simulink model "ModeAdjust"  (R2018b)
settings: Solver=FixedStepDiscrete  StartTime=0.0  StopTime=inf  FixedStep=0.01  RelTol=1e-3
undefined symbols (not defined in the file or in its folder): IfKeSMSbSeatMovBkRclnEnable_Val, IfKeSMSbSeatMovFrwdBkwdEnable_Val, IfKeSMSbSeatMovFtrstEnable_Val, IfKeSMSbSeatMovHdrstFrwdBkwdEnable_Val, IfKeSMSbSeatMovHdUpwdDnwdEnable_Val, IfKeSMSbSeatMovLgrstEnable_Val, IfKeSMSbSeatMovLtwdRtwdEnable_Val, IfVeSMSeStNumConfig, KeSMSbArmscreenMovEnable_Val, KeSMSbSeatMovLgrstExpdEnable_Val, KeSMSuFirstRwStBackPosDelta_Val, KeSMSuFirstRwStBackPosTolr_Val, KeSMSuFirstRwStCushFrntPosDelta_Val, KeSMSuFirstRwStCushFrntPosTolr_Val, KeSMSuFirstRwStCushRePosDelta_Val, KeSMSuFirstRwStCushRePosTolr_Val, KeSMSuFirstRwStFootrestPosDelta_Val, KeSMSuFirstRwStFootrestPosTolr_Val, KeSMSuFirstRwStFwdBkwdPosDelta_Val, KeSMSuFirstRwStFwdBkwdPosTolr_Val, KeSMSuMdMotFinshdTm_Val, KeSMSuMdRetryTm1_Val, KeSMSuModeReqDurgTm_Val, KeSMSuSecRwStArmTochPosDelta_Val, KeSMSuSecRwStArmTochPosTolr_Val, KeSMSuSecRwStBackPosDelta_Val, KeSMSuSecRwStBackPosTolr_Val, KeSMSuSecRwStFtrstUpwdDnwdPosDelta_Val, KeSMSuSecRwStFtrstUpwdDnwdPosTolr_Val, KeSMSuSecRwStFwdBkwdPosDelta_Val, KeSMSuSecRwStFwdBkwdPosTolr_Val, KeSMSuSecRwStHeadrestFwdBkwdPosDelta_Val, KeSMSuSecRwStHeadrestFwdBkwdPosTolr_Val, KeSMSuSecRwStHeadrestUpwdDwnwdPosDelta_Val, KeSMSuSecRwStHeadrestUpwdDwnwdPosTolr_Val, KeSMSuSecRwStLegrestInOutPosDelta_Val, KeSMSuSecRwStLegrestInOutPosTolr_Val, KeSMSuSecRwStLegrestUpwdDwnwdPosDelta_Val, KeSMSuSecRwStLegrestUpwdDwnwdPosTolr_Val, KeSMSuSecRwStLwdRwdPosDelta_Val, KeSMSuSecRwStLwdRwdPosTolr_Val, KeSMSuSecRwStVIPFtrstRefAngle_Val, KeSMSuThirdRwStFwdBkwdPosDelta_Val, KeSMSuThirdRwStFwdBkwdPosTolr_Val, KeSMSuThrdRwCushFoldPosDelta_Val, KeSMSuThrdRwCushFoldPosTolr_Val, KeSMSuThrdRwStBackPosDelta_Val, KeSMSuThrdRwStBackPosTolr_Val, KeSMSw4SLegrstCloseMdSecRwLtStFtrstUpwdDnwdPos_Val, KeSMSw4SLegrstCloseMdSecRwLtStFtrstUpwdDnwdPosMax_Val, KeSMSw4SLegrstCloseMdSecRwLtStFtrstUpwdDnwdPosMin_Val, KeSMSw4SLegrstCloseMdSecRwLtStLgrstOtwdInwdPos_Val, KeSMSw4SLegrstCloseMdSecRwLtStLgrstOtwdInwdPosMax_Val, KeSMSw4SLegrstCloseMdSecRwLtStLgrstOtwdInwdPosMin_Val, KeSMSw4SLegrstCloseMdSecRwLtStLgrstUpwdDnwdPos_Val, KeSMSw4SLegrstCloseMdSecRwLtStLgrstUpwdDnwdPosMax_Val, KeSMSw4SLegrstCloseMdSecRwLtStLgrstUpwdDnwdPosMin_Val, KeSMSw4SLegrstCloseMdSecRwRtStFtrstUpwdDnwdPos_Val, KeSMSw4SLegrstCloseMdSecRwRtStFtrstUpwdDnwdPosMax_Val, KeSMSw4SLegrstCloseMdSecRwRtStFtrstUpwdDnwdPosMin_Val ... (+1138)
libraries: Lib x401
(part 2 of 35)

== system ModeAdjust/ModeAdjustRunnable_sys ==
  IfVeSMSeSecRwLtStChldLkRsp_Val_read : Inport
  IfVeSMSeSecRwRtStChldLkRsp_Val_read : Inport  Port=2
  IfVeSMSuDrvStBkReclnUpwdDnwdPos_Val_read : Inport  Port=3
  IfVeSMSuDrvStBkReclnUpwdDnwdPosV_Val_read : Inport  Port=4
  IfVeSMSuDrvStCshnFrntUpwdDnwdPos_Val_read : Inport  Port=5
  IfVeSMSuDrvStCshnFrntUpwdDnwdPosV_Val_read : Inport  Port=6
  IfVeSMSuDrvStCshnRrUpwdDnwdPos_Val_read : Inport  Port=7
  IfVeSMSuDrvStCshnRrUpwdDnwdPosV_Val_read : Inport  Port=8
  IfVeSMSuDrvStFrwdBkwdPos_Val_read : Inport  Port=9
  IfVeSMSuDrvStFrwdBkwdPosV_Val_read : Inport  Port=10
  IfVeSMSuDrvStFtUpwdDnwdPos_Val_read : Inport  Port=11
  IfVeSMSuDrvStFtUpwdDnwdPosV_Val_read : Inport  Port=12
  IfVeSMSuPassStBkReclnUpwdDnwdPos_Val_read : Inport  Port=13
  IfVeSMSuPassStBkReclnUpwdDnwdPosV_Val_read : Inport  Port=14
  IfVeSMSuPassStCshnFrntUpwdDnwdPos_Val_read : Inport  Port=15
  IfVeSMSuPassStCshnFrntUpwdDnwdPosV_Val_read : Inport  Port=16
  IfVeSMSuPassStCshnRrUpwdDnwdPos_Val_read : Inport  Port=17
  IfVeSMSuPassStCshnRrUpwdDnwdPosV_Val_read : Inport  Port=18
  IfVeSMSuPassStFrwdBkwdPos_Val_read : Inport  Port=19
  IfVeSMSuPassStFrwdBkwdPosV_Val_read : Inport  Port=20
  IfVeSMSuPassStFtUpwdDnwdPos_Val_read : Inport  Port=21
  IfVeSMSuPassStFtUpwdDnwdPosV_Val_read : Inport  Port=22
  IfVeSMSuSecRwLtStArmScrnPos_Val_read : Inport  Port=23
  IfVeSMSuSecRwLtStArmScrnPosV_Val_read : Inport  Port=24
  IfVeSMSuSecRwLtStBkReclnUpwdDnwdPos_Val_read : Inport  Port=25
  IfVeSMSuSecRwLtStBkReclnUpwdDnwdPosV_Val_read : Inport  Port=26
  IfVeSMSuSecRwLtStFrwdBkwdPos_Val_read : Inport  Port=27
  IfVeSMSuSecRwLtStFrwdBkwdPosV_Val_read : Inport  Port=28
  IfVeSMSuSecRwLtStHdrstUpwdDnwdPos_Val_read : Inport  Port=29
  IfVeSMSuSecRwLtStHdrstUpwdDnwdPosV_Val_read : Inport  Port=30
  IfVeSMSuSecRwLtStLgrstUpwdDnwdPos_Val_read : Inport  Port=31
  IfVeSMSuSecRwLtStLgrstUpwdDnwdPosV_Val_read : Inport  Port=32
  IfVeSMSuSecRwLtStLtwdRtwdPos_Val_read : Inport  Port=33
  IfVeSMSuSecRwLtStLtwdRtwdPosV_Val_read : Inport  Port=34
  IfVeSMSuSecRwRtStArmScrnPos_Val_read : Inport  Port=35
  IfVeSMSuSecRwRtStArmScrnPosV_Val_read : Inport  Port=36
  IfVeSMSuSecRwRtStBkReclnUpwdDnwdPos_Val_read : Inport  Port=37
  IfVeSMSuSecRwRtStBkReclnUpwdDnwdPosV_Val_read : Inport  Port=38
  IfVeSMSuSecRwRtStFrwdBkwdPos_Val_read : Inport  Port=39
  IfVeSMSuSecRwRtStFrwdBkwdPosV_Val_read : Inport  Port=40
  IfVeSMSuSecRwRtStHdrstUpwdDnwdPos_Val_read : Inport  Port=41
  IfVeSMSuSecRwRtStHPassStUpwdDnwdPosV_Val_read : Inport  Port=42
  IfVeSMSuSecRwRtStLgrstUpwdDnwdPos_Val_read : Inport  Port=43
  IfVeSMSuSecRwRtStLgrstUpwdDnwdPosV_Val_read : Inport  Port=44
  IfVeSMSuSecRwRtStLtwdRtwdPos_Val_read : Inport  Port=45
  IfVeSMSuSecRwRtStLtwdRtwdPosV_Val_read : Inport  Port=46
  IfVeSMSuThdRwLtStBkReclnUpwdDnwdPos_Val_read : Inport  Port=47
  IfVeSMSuThdRwLtStBkReclnUpwdDnwdPosV_Val_read : Inport  Port=48
  IfVeSMSuThdRwLtStCshnFldUpwdDnwdPos_Val_read : Inport  Port=49
  IfVeSMSuThdRwLtStCshnFldUpwdDnwdPosV_Val_read : Inport  Port=50
  IfVeSMSuThdRwLtStFrwdBkwdPos_Val_read : Inport  Port=51
  IfVeSMSuThdRwLtStFrwdBkwdPosV_Val_read : Inport  Port=52
  IfVeSMSuThdRwRStFrwdBkwdPos_Val_read : Inport  Port=53
  IfVeSMSuThdRwRtStBkReclnUpwdDnwdPos_Val_read : Inport  Port=54
  IfVeSMSuThdRwRtStBkReclnUpwdDnwdPosV_Val_read : Inport  Port=55
  IfVeSMSuThdRwRtStCshnFldUpwdDnwdPos_Val_read : Inport  Port=56
  IfVeSMSuThdRwRtStCshnFldUpwdDnwdPosV_Val_read : Inport  Port=57
  IfVeSMSuThdRwRtStFrwdBkwdPosV_Val_read : Inport  Port=58
  IfVeSMSeNotThdRowRtSeaOccStat_Val_read : Inport  Port=59
  IfVeSMSeNotThdRwCtStOccStat_Val_read : Inport  Port=60
  IfVeSMSeNotThdRwLtStOccStat_Val_read : Inport  Port=61
  modestate32_Val_read : Inport  Port=62
  PwrMdChked_Val_read : Inport  Port=63
  IfVeSMSbDrvStBkReclnUpwdDnwdMovConfig_Val_read : Inport  Port=64
  IfVeSMSbDrvStFrwdBkwdMovConfig_Val_read : Inport  Port=65
  IfVeSMSbDrvStFtUpwdDnwdMovConfig_Val_read : Inport  Port=66
  IfVeSMSbPassStBkReclnUpwdDnwdMovConfig_Val_read : Inport  Port=67
  IfVeSMSbPassStFrwdBkwdMovConfig_Val_read : Inport  Port=68
  IfVeSMSbPassStFtUpwdDnwdMovConfig_Val_read : Inport  Port=69
  IfVeSMSbSecRwRtStBkReclnUpwdDnwdMovConfig_Val_read : Inport  Port=70
  IfVeSMSbSecRwRtStBlstOtwdInwdMovConfig_Val_read : Inport  Port=71
  IfVeSMSbSecRwRtStFrwdBkwdMovConfig_Val_read : Inport  Port=72
  IfVeSMSbSecRwRtStLgrstUpwdMovConfig_Val_read : Inport  Port=73
  IfVeSMSbSecRwRtStLtwdRtwdMovConfig_Val_read : Inport  Port=74
  IfVeSMSbThdRwLtStBkReclnUpwdDnwdMovConfig_Val_read : Inport  Port=75
  IfVeSMSbThdRwLtStCshnFldUpwdDnwdMovConfig_Val_read : Inport  Port=76
  IfVeSMSbThdRwLtStFrwdBkwdMovConfig_Val_read : Inport  Port=77
  IfVeSMSbThdRwRtStBkReclnUpwdDnwdMovConfig_Val_read : Inport  Port=78
  IfVeSMSbThdRwRtStCshnFldUpwdDnwdMovConfig_Val_read : Inport  Port=79
  IfVeSMSbThdRwRtStFrwdBkwdMovConfig_Val_read : Inport  Port=80
  IfVeSMSuRrLtStFtUpwdDnwdPos_Val_read : Inport  Port=81
  IfVeSMSuRrLtStFtUpwdDnwdPosV_Val_read : Inport  Port=82
  IfVeSMSuRrRtStFtUpwdDnwdPos_Val_read : Inport  Port=83
  IfVeSMSuRrRtStFtUpwdDnwdPosV_Val_read : Inport  Port=84
  IfVeSMSuSecRwLtStLgrstOtwdInwdPos_Val_read : Inport  Port=85
  IfVeSMSuSecRwLtStLgrstOtwdInwdPosV_Val_read : Inport  Port=86
  IfVeSMSuSecRwRtStLgrstOtwdInwdPos_Val_read : Inport  Port=87
  IfVeSMSuSecRwRtStLgrstOtwdInwdPosV_Val_read : Inport  Port=88
  IfVeSMSbSecRwRtSLgrstExpdMovConfig_Val_read : Inport  Port=89
  IfVeSMSbSecRwRtStFtrstMovConfig_Val_read : Inport  Port=90
  IfVeSMSbSecRwRtStHdUpwdDnwdMovConfig_Val_read : Inport  Port=91
  IfVeSMSbThdRwLtStFrwdCmdSrv_Val_read : Inport  Port=92
  IfVeSMSbThdRwRtStFrwdCmdSrv_Val_read : Inport  Port=93
  IfVeSMSbSecRwRtStHdrstFrwdBkwdMovConfig_Val_read : Inport  Port=94
  IfVeSMSuSecRwLtStHdrstFrwdBkwdPos_Val_read : Inport  Port=95
  IfVeSMSuSecRwLtStHdrstFrwdBkwdPosV_Val_read : Inport  Port=96
  IfVeSMSuSecRwRtStHdrstFrwdBkwdPos_Val_read : Inport  Port=97
  IfVeSMSuSecRwRtStHdrstFrwdBkwdPosV_Val_read : Inport  Port=98
  IfVeSMSeNotSecRowLeSeaOccStat_Val_read : Inport  Port=99
  IfVeSMSeNotSecRowRtSeaOccStat_Val_read : Inport  Port=100
  IfVeSMSeStNumConfig_Val_read : Inport  Port=101
  function : TriggerPort  TriggerType=function-call  VariantControl=(inherit)  SampleTimeType=periodic  SampleTime=-1
  ModeAdjust : Subsystem
  IfVeSMSbDrvStRclCmdSrv_Val_write : Outport
  IfVeSMSbSecRwRtStRclCmdSrv_Val_write : Outport  Port=2
  IfVeSMSbThdRwLtStRclCmdSrv_Val_write : Outport  Port=3
  IfVeSMSbThdRwRtStRclCmdSrv_Val_write : Outport  Port=4
  IfVeSMSuDrvStBkReclnUpwdDnwdTrgtPos_Val_write : Outport  Port=5
  IfVeSMSuDrvStCshnFrntUpwdDnwdTrgtPos_Val_write : Outport  Port=6
  IfVeSMSuDrvStCshnRrUpwdDnwdTrgtPos_Val_write : Outport  Port=7
  IfVeSMSuDrvStFrwdBkwdTrgtPos_Val_write : Outport  Port=8
  IfVeSMSuDrvStFtUpwdDnwdTrgtPos_Val_write : Outport  Port=9
  IfVeSMSuPassStBkReclnUpwdDnwdTrgtPos_Val_write : Outport  Port=10
  IfVeSMSuPassStCshnFrntUpwdDnwdTrgtPos_Val_write : Outport  Port=11
  IfVeSMSuPassStCshnRrUpwdDnwdTrgtPos_Val_write : Outport  Port=12
  IfVeSMSuPassStFrwdBkwdTrgtPos_Val_write : Outport  Port=13
  IfVeSMSuPassStFtUpwdDnwdTrgtPos_Val_write : Outport  Port=14
  IfVeSMSuPassStRclCmdSrv_Val_write : Outport  Port=15
  IfVeSMSuSecRwLtStBkReclnUpwdDnwdTrgtPos_Val_write : Outport  Port=16
  IfVeSMSuSecRwLtStFrwdBkwdTrgtPos_Val_write : Outport  Port=17
  IfVeSMSuSecRwLtStHdrstUpwdDnwdTrgtPos_Val_write : Outport  Port=18
  IfVeSMSuSecRwLtStLgrstUpwdDnwdTrgtPos_Val_write : Outport  Port=19
  IfVeSMSuSecRwLtStLtwdRtwdTrgtPos_Val_write : Outport  Port=20
  IfVeSMSuSecRwLtStRclCmdSrv_Val_write : Outport  Port=21
  IfVeSMSuSecRwRtStBkReclnUpwdDnwdTrgtPos_Val_write : Outport  Port=22
  IfVeSMSuSecRwRtStFrwdBkwdTrgtPos_Val_write : Outport  Port=23
  IfVeSMSuSecRwRtStHdrstUpwdDnwdTrgtPos_Val_write : Outport  Port=24
  IfVeSMSuSecRwRtStLgrstUpwdDnwdTrgtPos_Val_write : Outport  Port=25
  IfVeSMSuSecRwRtStLtwdRtwdTrgtPos_Val_write : Outport  Port=26
  IfVeSMSuThdRwLtStBkReclnUpwdDnwdTrgtPos_Val_write : Outport  Port=27
  IfVeSMSuThdRwLtStCshnFldUpwdDnwdTrgtPos_Val_write : Outport  Port=28
  IfVeSMSuThdRwLtStFrwdBkwdTrgtPos_Val_write : Outport  Port=29
  IfVeSMSuThdRwRtStBkReclnUpwdDnwdTrgtPos_Val_write : Outport  Port=30
  IfVeSMSuThdRwRtStCshnFldUpwdDnwdTrgtPos_Val_write : Outport  Port=31
  IfVeSMSuThdRwRtStFrwdBkwdTrgtPos_Val_write : Outport  Port=32
  isAcsMdEntryArrivedAtTargetPos_Val_write : Outport  Port=33
  isAcsMdEntryDoneFailed_Val_write : Outport  Port=34
  isAcsMdEntryDoneOK_Val_write : Outport  Port=35
  isAcsMdExtArrivedAtTargetPos_Val_write : Outport  Port=36
  isAcsMdExtDoneFailed_Val_write : Outport  Port=37
  isAcsMdExtDoneOK_Val_write : Outport  Port=38
  isLfLugArrivedAtTargetPos_Val_write : Outport  Port=39
  isLfLugDoneFailed_Val_write : Outport  Port=40
  isLfLugDoneOK_Val_write : Outport  Port=41
  isLfRecoveryArrivedAtTargetPos_Val_write : Outport  Port=42
  isLfRecoveryDoneFailed_Val_write : Outport  Port=43
  isLfRecoveryDoneOK_Val_write : Outport  Port=44
  isLfVipArrivedAtTargetPos_Val_write : Outport  Port=45
  isLfVipDoneFailed_Val_write : Outport  Port=46
  isLfVipDoneOK_Val_write : Outport  Port=47
  isRtLugArrivedAtTargetPos_Val_write : Outport  Port=48
  isRtLugDoneFailed_Val_write : Outport  Port=49
  isRtLugDoneOK_Val_write : Outport  Port=50
  isRtRecoveryArrivedAtTargetPos_Val_write : Outport  Port=51
  isRtRecoveryDoneFailed_Val_write : Outport  Port=52
  isRtRecoveryDoneOK_Val_write : Outport  Port=53
  isRtVipArrivedAtTargetPos_Val_write : Outport  Port=54
  isRtVipDoneFailed_Val_write : Outport  Port=55
  isRtVipDoneOK_Val_write : Outport  Port=56
  IfVeSMSuSecRwLtStArmScrnTrgtPos_Val_write : Outport  Port=57
  IfVeSMSuSecRwRtStArmScrnTrgtPos_Val_write : Outport  Port=58
  IfVeSMSuRrLtStFtUpwdDnwdTrgtPos_Val_write : Outport  Port=59
      settings: EnsureOutportIsVirtual=on
  IfVeSMSuRrRtStFtUpwdDnwdTrgtPos_Val_write : Outport  Port=60
      settings: EnsureOutportIsVirtual=on
  IfVeSMSuSecRwLtStLgrstOtwdInwdTrgtPos_Val_write : Outport  Port=61
      settings: EnsureOutportIsVirtual=on
  IfVeSMSuSecRwRtStLgrstOtwdInwdTrgtPos_Val_write : Outport  Port=62
      settings: EnsureOutportIsVirtual=on
  isINTMArrivedAtTargetPos_Val_write : Outport  Port=63
      settings: EnsureOutportIsVirtual=on
  isINTMDoneFailed_Val_write : Outport  Port=64
      settings: EnsureOutportIsVirtual=on
  isINTMDoneOK_Val_write : Outport  Port=65
      settings: EnsureOutportIsVirtual=on
  isLfFamlyArrivedAtTargetPos_Val_write : Outport  Port=66
      settings: EnsureOutportIsVirtual=on
  isLfFamlyDoneFailed_Val_write : Outport  Port=67
      settings: EnsureOutportIsVirtual=on
  isLfFamlyDoneOK_Val_write : Outport  Port=68
      settings: EnsureOutportIsVirtual=on
  isLfLyArrivedAtTargetPos_Val_write : Outport  Port=69
      settings: EnsureOutportIsVirtual=on
  isLfLyDoneFailed_Val_write : Outport  Port=70
      settings: EnsureOutportIsVirtual=on
  isLfLyDoneOK_Val_write : Outport  Port=71
      settings: EnsureOutportIsVirtual=on
  isRfFamlyDoneFailed_Val_write : Outport  Port=72
      settings: EnsureOutportIsVirtual=on
  isRfFamlyDoneOK_Val_write : Outport  Port=73
      settings: EnsureOutportIsVirtual=on
  isRtFamlyArrivedAtTargetPos_Val_write : Outport  Port=74
      settings: EnsureOutportIsVirtual=on
  isRtLyArrivedAtTargetPos_Val_write : Outport  Port=75
      settings: EnsureOutportIsVirtual=on
  isRtLyDoneFailed_Val_write : Outport  Port=76
      settings: EnsureOutportIsVirtual=on
  isRtLyDoneOK_Val_write : Outport  Port=77
      settings: EnsureOutportIsVirtual=on
  IfVeSMSuSecRwLtStHdrstFrwdBkwdTrgtPos_Val_write : Outport  Port=78
      settings: EnsureOutportIsVirtual=on
  IfVeSMSuSecRwRtStHdrstFrwdBkwdTrgtPos_Val_write : Outport  Port=79
      settings: EnsureOutportIsVirtual=on
  IfVeSMSeSecRwLtStMdRclLgSldSpdCrl_Val_write : Outport  Port=80
      settings: EnsureOutportIsVirtual=on
  IfVeSMSeSecRwRtStMdRclLgSldSpdCrl_Val_write : Outport  Port=81
      settings: EnsureOutportIsVirtual=on
  IfVeSMSeThdRwLtStMdRclLgSldSpdCrl_Val_write : Outport  Port=82
      settings: EnsureOutportIsVirtual=on
  IfVeSMSeThdRwRtStMdRclLgSldSpdCrl_Val_write : Outport  Port=83
      settings: EnsureOutportIsVirtual=on
  isINTMRArrivedAtTargetPos_Val_write : Outport  Port=84
      settings: EnsureOutportIsVirtual=on
  isINTMRDoneFailed_Val_write : Outport  Port=85
      settings: EnsureOutportIsVirtual=on
  isINTMRDoneOK_Val_write : Outport  Port=86
      settings: EnsureOutportIsVirtual=on
  isLgrstCloseLArrivedAtTargetPos_Val_write : Outport  Port=87
      settings: EnsureOutportIsVirtual=on
  isLgrstCloseLDoneFailed_Val_write : Outport  Port=88
      settings: EnsureOutportIsVirtual=on
  isLgrstCloseLDoneOK_Val_write : Outport  Port=89
      settings: EnsureOutportIsVirtual=on
  isLgrstCloseRArrivedAtTargetPos_Val_write : Outport  Port=90
      settings: EnsureOutportIsVirtual=on
  isLgrstCloseRDoneFailed_Val_write : Outport  Port=91
      settings: EnsureOutportIsVirtual=on
  isLgrstCloseRDoneOK_Val_write : Outport  Port=92
      settings: EnsureOutportIsVirtual=on
  isLgrstOpenLArrivedAtTargetPos_Val_write : Outport  Port=93
      settings: EnsureOutportIsVirtual=on
  isLgrstOpenLDoneFailed_Val_write : Outport  Port=94
      settings: EnsureOutportIsVirtual=on
  isLgrstOpenLDoneOK_Val_write : Outport  Port=95
      settings: EnsureOutportIsVirtual=on
  isLgrstOpenRArrivedAtTargetPos_Val_write : Outport  Port=96
      settings: EnsureOutportIsVirtual=on
  isLgrstOpenRDoneFailed_Val_write : Outport  Port=97
      settings: EnsureOutportIsVirtual=on
  isLgrstOpenRDoneOK_Val_write : Outport  Port=98
      settings: EnsureOutportIsVirtual=on
  wires:
  IfVeSMSuPassStBkReclnUpwdDnwdPos_Val_read/1 -> ModeAdjust/3(IfVeSMSuPassStBkReclnUpwdDnwdPos_Val_read)
  IfVeSMSuPassStBkReclnUpwdDnwdPosV_Val_read/1 -> ModeAdjust/4(IfVeSMSuPassStBkReclnUpwdDnwdPosV_Val_read)
  IfVeSMSuPassStCshnFrntUpwdDnwdPos_Val_read/1 -> ModeAdjust/5(IfVeSMSuPassStCshnFrntUpwdDnwdPos_Val_read)
  IfVeSMSuPassStCshnFrntUpwdDnwdPosV_Val_read/1 -> ModeAdjust/6(IfVeSMSuPassStCshnFrntUpwdDnwdPosV_Val_read)
  IfVeSMSuPassStCshnRrUpwdDnwdPos_Val_read/1 -> ModeAdjust/7(IfVeSMSuPassStCshnRrUpwdDnwdPos_Val_read)
  IfVeSMSuPassStCshnRrUpwdDnwdPosV_Val_read/1 -> ModeAdjust/8(IfVeSMSuPassStCshnRrUpwdDnwdPosV_Val_read)
  IfVeSMSuPassStFrwdBkwdPos_Val_read/1 -> ModeAdjust/9(IfVeSMSuPassStFrwdBkwdPos_Val_read)
  IfVeSMSuPassStFrwdBkwdPosV_Val_read/1 -> ModeAdjust/10(IfVeSMSuPassStFrwdBkwdPosV_Val_read)
  IfVeSMSuPassStFtUpwdDnwdPos_Val_read/1 -> ModeAdjust/11(IfVeSMSuPassStFtUpwdDnwdPos_Val_read)
  IfVeSMSuPassStFtUpwdDnwdPosV_Val_read/1 -> ModeAdjust/12(IfVeSMSuPassStFtUpwdDnwdPosV_Val_read)
  IfVeSMSuSecRwLtStArmScrnPos_Val_read/1 -> ModeAdjust/58(IfVeSMSuSecRwLtStArmScrnPos_Val_read)
  IfVeSMSuSecRwLtStArmScrnPosV_Val_read/1 -> ModeAdjust/59(IfVeSMSuSecRwLtStArmScrnPosV_Val_read)
  IfVeSMSuSecRwLtStBkReclnUpwdDnwdPos_Val_read/1 -> ModeAdjust/13(IfVeSMSuSecRwLtStBkReclnUpwdDnwdPos_Val_read)
  IfVeSMSuSecRwLtStBkReclnUpwdDnwdPosV_Val_read/1 -> ModeAdjust/14(IfVeSMSuSecRwLtStBkReclnUpwdDnwdPosV_Val_read)
  IfVeSMSuSecRwLtStFrwdBkwdPos_Val_read/1 -> ModeAdjust/15(IfVeSMSuSecRwLtStFrwdBkwdPos_Val_read)
  IfVeSMSuSecRwLtStFrwdBkwdPosV_Val_read/1 -> ModeAdjust/16(IfVeSMSuSecRwLtStFrwdBkwdPosV_Val_read)
  IfVeSMSuSecRwLtStLgrstUpwdDnwdPos_Val_read/1 -> ModeAdjust/19(IfVeSMSuSecRwLtStLgrstUpwdDnwdPos_Val_read)
  IfVeSMSuSecRwLtStLgrstUpwdDnwdPosV_Val_read/1 -> ModeAdjust/20(IfVeSMSuSecRwLtStLgrstUpwdDnwdPosV_Val_read)
  IfVeSMSuSecRwLtStLtwdRtwdPos_Val_read/1 -> ModeAdjust/21(IfVeSMSuSecRwLtStLtwdRtwdPos_Val_read)
  IfVeSMSuSecRwLtStLtwdRtwdPosV_Val_read/1 -> ModeAdjust/22(IfVeSMSuSecRwLtStLtwdRtwdPosV_Val_read)
  IfVeSMSuSecRwRtStArmScrnPos_Val_read/1 -> ModeAdjust/60(SecRwRtStArmScrnPos_Val_read)
  IfVeSMSuSecRwRtStArmScrnPosV_Val_read/1 -> ModeAdjust/61(SecRwRtStArmScrnPosV_Val_read)
  IfVeSMSuSecRwRtStBkReclnUpwdDnwdPos_Val_read/1 -> ModeAdjust/35(IfVeSMSuSecRwRtStBkReclnUpwdDnwdPos_Val_read)
  IfVeSMSuSecRwRtStBkReclnUpwdDnwdPosV_Val_read/1 -> ModeAdjust/36(IfVeSMSuSecRwRtStBkReclnUpwdDnwdPosV_Val_read)
  IfVeSMSuSecRwRtStFrwdBkwdPos_Val_read/1 -> ModeAdjust/37(IfVeSMSuSecRwRtStFrwdBkwdPos_Val_read)
  IfVeSMSuSecRwRtStFrwdBkwdPosV_Val_read/1 -> ModeAdjust/38(IfVeSMSuSecRwRtStFrwdBkwdPosV_Val_read)
  IfVeSMSuSecRwRtStHdrstUpwdDnwdPos_Val_read/1 -> ModeAdjust/39(IfVeSMSuSecRwRtStHPassStUpwdDnwdPos_Val_read)
  IfVeSMSuSecRwRtStHPassStUpwdDnwdPosV_Val_read/1 -> ModeAdjust/40(IfVeSMSuSecRwRtStHPassStUpwdDnwdPosV_Val_read)
  IfVeSMSuSecRwRtStLgrstUpwdDnwdPos_Val_read/1 -> ModeAdjust/41(IfVeSMSuSecRwRtStLgrstUpwdDnwdPos_Val_read)
  IfVeSMSuSecRwRtStLgrstUpwdDnwdPosV_Val_read/1 -> ModeAdjust/42(IfVeSMSuSecRwRtStLgrstUpwdDnwdPosV_Val_read)
  IfVeSMSuSecRwRtStLtwdRtwdPos_Val_read/1 -> ModeAdjust/43(IfVeSMSuSecRwRtStLtwdRtwdPos_Val_read)
  IfVeSMSuSecRwRtStLtwdRtwdPosV_Val_read/1 -> ModeAdjust/44(IfVeSMSuSecRwRtStLtwdRtwdPosV_Val_read)
  IfVeSMSuThdRwLtStBkReclnUpwdDnwdPos_Val_read/1 -> ModeAdjust/23(IfVeSMSuThdRwLtStBkReclnUpwdDnwdPos_Val_read)
  IfVeSMSuThdRwLtStBkReclnUpwdDnwdPosV_Val_read/1 -> ModeAdjust/24(IfVeSMSuThdRwLtStBkReclnUpwdDnwdPosV_Val_read)
  IfVeSMSuThdRwLtStCshnFldUpwdDnwdPos_Val_read/1 -> ModeAdjust/25(IfVeSMSuThdRwLtStCshnFldUpwdDnwdPos_Val_read)
  IfVeSMSuThdRwLtStCshnFldUpwdDnwdPosV_Val_read/1 -> ModeAdjust/26(IfVeSMSuThdRwLtStCshnFldUpwdDnwdPosV_Val_read)
  IfVeSMSuThdRwLtStFrwdBkwdPos_Val_read/1 -> ModeAdjust/27(IfVeSMSuThdRwLtStFrwdBkwdPos_Val_read)
  IfVeSMSuThdRwLtStFrwdBkwdPosV_Val_read/1 -> ModeAdjust/28(IfVeSMSuThdRwLtStFrwdBkwdPosV_Val_read)
  IfVeSMSuThdRwRStFrwdBkwdPos_Val_read/1 -> ModeAdjust/33(IfVeSMSuThdRwRtStFrwdBkwdPos_Val_read)
  IfVeSMSuThdRwRtStBkReclnUpwdDnwdPos_Val_read/1 -> ModeAdjust/29(IfVeSMSuThdRwRtStBkReclnUpwdDnwdPos_Val_read)
  IfVeSMSuThdRwRtStBkReclnUpwdDnwdPosV_Val_read/1 -> ModeAdjust/30(IfVeSMSuThdRwRtStBkReclnUpwdDnwdPosV_Val_read)
  IfVeSMSuThdRwRtStCshnFldUpwdDnwdPos_Val_read/1 -> ModeAdjust/31(IfVeSMSuThdRwRtStCshnFldUpwdDnwdPos_Val_read)
  IfVeSMSuThdRwRtStCshnFldUpwdDnwdPosV_Val_read/1 -> ModeAdjust/32(IfVeSMSuThdRwRtStCshnFldUpwdDnwdPosV_Val_read)
  IfVeSMSuThdRwRtStFrwdBkwdPosV_Val_read/1 -> ModeAdjust/34(IfVeSMSuThdRwRtStFrwdBkwdPosV_Val_read)
  ModeAdjust/32(IfVeSMSbDrvStRclCmdSrv_Val_write) -> IfVeSMSbDrvStRclCmdSrv_Val_write/1
  ModeAdjust/29(IfVeSMSbSecRwRtStRclCmdSrv_Val_write) -> IfVeSMSbSecRwRtStRclCmdSrv_Val_write/1
  ModeAdjust/28(IfVeSMSbThdRwLtStRclCmdSrv_Val_write) -> IfVeSMSbThdRwLtStRclCmdSrv_Val_write/1
  ModeAdjust/27(IfVeSMSbThdRwRtStRclCmdSrv_Val_write) -> IfVeSMSbThdRwRtStRclCmdSrv_Val_write/1
  ModeAdjust/9(DrvStBkReclnUpwdDnwdTrgtPos) -> IfVeSMSuDrvStBkReclnUpwdDnwdTrgtPos_Val_write/1
  ModeAdjust/11(DrvStCshnFrntUpwdDnwdTrgtPos) -> IfVeSMSuDrvStCshnFrntUpwdDnwdTrgtPos_Val_write/1
  ModeAdjust/13(DrvStCshnRrUpwdDnwdTrgtPos) -> IfVeSMSuDrvStCshnRrUpwdDnwdTrgtPos_Val_write/1
  ModeAdjust/15(DrvStFrwdBkwdTrgtPos) -> IfVeSMSuDrvStFrwdBkwdTrgtPos_Val_write/1
  ModeAdjust/4(DrvStFtUpwdDnwdTrgtPos) -> IfVeSMSuDrvStFtUpwdDnwdTrgtPos_Val_write/1
  ModeAdjust/20(PassStBkReclnUpwdDnwdTrgtPos) -> IfVeSMSuPassStBkReclnUpwdDnwdTrgtPos_Val_write/1
  ModeAdjust/23(PassStCshnFrntUpwdDnwdTrgtPos) -> IfVeSMSuPassStCshnFrntUpwdDnwdTrgtPos_Val_write/1
  ModeAdjust/24(PassStCshnRrUpwdDnwdTrgtPos) -> IfVeSMSuPassStCshnRrUpwdDnwdTrgtPos_Val_write/1
  ModeAdjust/25(PassStFrwdBkwdTrgtPos) -> IfVeSMSuPassStFrwdBkwdTrgtPos_Val_write/1
  ModeAdjust/26(PassStFtUpwdDnwdTrgtPos) -> IfVeSMSuPassStFtUpwdDnwdTrgtPos_Val_write/1
  ModeAdjust/33(IfVeSMSuPassStRclCmdSrv_Val_write) -> IfVeSMSuPassStRclCmdSrv_Val_write/1
  ModeAdjust/30(SecRwLtStBkReclnUpwdDnwdTrgtPos) -> IfVeSMSuSecRwLtStBkReclnUpwdDnwdTrgtPos_Val_write/1
  ModeAdjust/34(SecRwLtStFrwdBkwdTrgtPos) -> IfVeSMSuSecRwLtStFrwdBkwdTrgtPos_Val_write/1
  ModeAdjust/35(SecRwLtStHdrstUpwdDnwdTrgtPos) -> IfVeSMSuSecRwLtStHdrstUpwdDnwdTrgtPos_Val_write/1
  ModeAdjust/36(SecRwLtStLgrstUpwdDnwdTrgtPos) -> IfVeSMSuSecRwLtStLgrstUpwdDnwdTrgtPos_Val_write/1
  ModeAdjust/37(SecRwLtStLtwdRtwdTrgtPos) -> IfVeSMSuSecRwLtStLtwdRtwdTrgtPos_Val_write/1
  ModeAdjust/31(IfVeSMSuSecRwLtStRclCmdSrv_Val_write) -> IfVeSMSuSecRwLtStRclCmdSrv_Val_write/1
  ModeAdjust/38(SecRwRtStBkReclnUpwdDnwdTrgtPos) -> IfVeSMSuSecRwRtStBkReclnUpwdDnwdTrgtPos_Val_write/1
  ModeAdjust/39(SecRwRtStFrwdBkwdTrgtPos) -> IfVeSMSuSecRwRtStFrwdBkwdTrgtPos_Val_write/1
  ModeAdjust/40(SecRwRtStHdrstUpwdDnwdTrgtPos) -> IfVeSMSuSecRwRtStHdrstUpwdDnwdTrgtPos_Val_write/1
  ModeAdjust/41(SecRwRtStLgrstUpwdDnwdTrgtPos) -> IfVeSMSuSecRwRtStLgrstUpwdDnwdTrgtPos_Val_write/1
  ModeAdjust/42(SecRwRtStLtwdRtwdTrgtPos) -> IfVeSMSuSecRwRtStLtwdRtwdTrgtPos_Val_write/1
  ModeAdjust/43(ThdRwLtStBkReclnUpwdDnwdTrgtPos) -> IfVeSMSuThdRwLtStBkReclnUpwdDnwdTrgtPos_Val_write/1
  ModeAdjust/44(ThdRwLtStCshnFldUpwdDnwdTrgtPos) -> IfVeSMSuThdRwLtStCshnFldUpwdDnwdTrgtPos_Val_write/1
  ModeAdjust/45(ThdRwLtStFrwdBkwdTrgtPos) -> IfVeSMSuThdRwLtStFrwdBkwdTrgtPos_Val_write/1
  ModeAdjust/46(ThdRwRtStBkReclnUpwdDnwdTrgtPos) -> IfVeSMSuThdRwRtStBkReclnUpwdDnwdTrgtPos_Val_write/1
  ModeAdjust/47(ThdRwRtStCshnFldUpwdDnwdTrgtPos) -> IfVeSMSuThdRwRtStCshnFldUpwdDnwdTrgtPos_Val_write/1
  ModeAdjust/48(ThdRwRtStFrwdBkwdTrgtPos) -> IfVeSMSuThdRwRtStFrwdBkwdTrgtPos_Val_write/1
  ModeAdjust/49(isAcsMdEntryArrivedAtTargetPos) -> isAcsMdEntryArrivedAtTargetPos_Val_write/1
  ModeAdjust/2(isAcsMdEntryDoneFailed) -> isAcsMdEntryDoneFailed_Val_write/1
  IfVeSMSuDrvStFtUpwdDnwdPos_Val_read/1 -> ModeAdjust/1(IfVeSMSuDrvStFtUpwdDnwdPos_Val_read)
  IfVeSMSuDrvStFtUpwdDnwdPosV_Val_read/1 -> ModeAdjust/2(IfVeSMSuDrvStFtUpwdDnwdPosV_Val_read)
  IfVeSMSuDrvStBkReclnUpwdDnwdPos_Val_read/1 -> ModeAdjust/45(IfVeSMSuDrvStBkReclnUpwdDnwdPos_Val_read)
  IfVeSMSuDrvStBkReclnUpwdDnwdPosV_Val_read/1 -> ModeAdjust/46(IfVeSMSuDrvStBkReclnUpwdDnwdPosV_Val_read)
  IfVeSMSuDrvStCshnFrntUpwdDnwdPos_Val_read/1 -> ModeAdjust/47(IfVeSMSuDrvStCshnFrntUpwdDnwdPos_Val_read)
  IfVeSMSuDrvStCshnFrntUpwdDnwdPosV_Val_read/1 -> ModeAdjust/48(IfVeSMSuDrvStCshnFrntUpwdDnwdPosV_Val_read)
  IfVeSMSuDrvStCshnRrUpwdDnwdPos_Val_read/1 -> ModeAdjust/49(IfVeSMSuDrvStCshnRrUpwdDnwdPos_Val_read)
  IfVeSMSuDrvStCshnRrUpwdDnwdPosV_Val_read/1 -> ModeAdjust/50(IfVeSMSuDrvStCshnRrUpwdDnwdPosV_Val_read)
  IfVeSMSuDrvStFrwdBkwdPos_Val_read/1 -> ModeAdjust/51(IfVeSMSuDrvStFrwdBkwdPos_Val_read)
  IfVeSMSuDrvStFrwdBkwdPosV_Val_read/1 -> ModeAdjust/52(IfVeSMSuDrvStFrwdBkwdPosV_Val_read)
  IfVeSMSeSecRwRtStChldLkRsp_Val_read/1 -> ModeAdjust/57(SecRwRtStChldLkRsp_R)
  IfVeSMSeSecRwLtStChldLkRsp_Val_read/1 -> ModeAdjust/56(SecRwRtStChldLkRsp_L)
  ModeAdjust/1(isAcsMdEntryDoneOK) -> isAcsMdEntryDoneOK_Val_write/1
  ModeAdjust/3(isAcsMdExtDoneOK) -> isAcsMdExtDoneOK_Val_write/1
  ModeAdjust/5(isAcsMdExtDoneFailed) -> isAcsMdExtDoneFailed_Val_write/1
  ModeAdjust/6(isLfVipDoneOK) -> isLfVipDoneOK_Val_write/1
  ModeAdjust/7(isLfVipDoneFailed) -> isLfVipDoneFailed_Val_write/1
  ModeAdjust/8(isRtVipDoneOK) -> isRtVipDoneOK_Val_write/1
  ModeAdjust/10(isRtVipDoneFailed) -> isRtVipDoneFailed_Val_write/1
  ModeAdjust/12(isLfRecoveryDoneOK) -> isLfRecoveryDoneOK_Val_write/1
  ModeAdjust/14(isLfRecoveryDoneFailed) -> isLfRecoveryDoneFailed_Val_write/1
  ModeAdjust/16(isRfRecoveryDoneOK) -> isRtRecoveryDoneOK_Val_write/1
  ModeAdjust/17(isRfRecoveryDoneFailed) -> isRtRecoveryDoneFailed_Val_write/1
  ModeAdjust/18(isLfLugDoneOK) -> isLfLugDoneOK_Val_write/1
  ModeAdjust/19(isLfLugDoneFailed) -> isLfLugDoneFailed_Val_write/1
  ModeAdjust/21(isRtLugDoneOK) -> isRtLugDoneOK_Val_write/1
  ModeAdjust/22(isRtLugDoneFailed) -> isRtLugDoneFailed_Val_write/1
  ModeAdjust/51(isLfVipArrivedAtTargetPos) -> isLfVipArrivedAtTargetPos_Val_write/1
  ModeAdjust/52(isRtVipArrivedAtTargetPos) -> isRtVipArrivedAtTargetPos_Val_write/1
  ModeAdjust/55(isLfRecoveryArrivedAtTargetPos) -> isLfRecoveryArrivedAtTargetPos_Val_write/1
  ModeAdjust/54(isRtLugArrivedAtTargetPos) -> isRtLugArrivedAtTargetPos_Val_write/1
  ModeAdjust/50(isAcsMdExtArrivedAtTargetPos) -> isAcsMdExtArrivedAtTargetPos_Val_write/1
  ModeAdjust/53(isLfLugArrivedAtTargetPos) -> isLfLugArrivedAtTargetPos_Val_write/1
  IfVeSMSuSecRwLtStHdrstUpwdDnwdPos_Val_read/1 -> ModeAdjust/17(IfVeSMSuSecRwLtStHPassStUpwdDnwdPos_Val_read)
  IfVeSMSuSecRwLtStHdrstUpwdDnwdPosV_Val_read/1 -> ModeAdjust/18(IfVeSMSuSecRwLtStHPassStUpwdDnwdPosV_Val_read)
  ModeAdjust/56(isRtRecoveryArrivedAtTargetPos) -> isRtRecoveryArrivedAtTargetPos_Val_write/1
  IfVeSMSeNotThdRwCtStOccStat_Val_read/1 -> ModeAdjust/53(IfVeSMSeNotThdRwCtStOccStatMSMSrc_Val_read)
  IfVeSMSeNotThdRwLtStOccStat_Val_read/1 -> ModeAdjust/54(IfVeSMSeNotThdRwLtStOccStatMSMSrc_Val_read)
  IfVeSMSeNotThdRowRtSeaOccStat_Val_read/1 -> ModeAdjust/55(IfVeSMSeNotThdRwRtStOccStatMSMSrc_Val_read)
  ModeAdjust/57(SecRwLtStArmScrnTrgtPos) -> IfVeSMSuSecRwLtStArmScrnTrgtPos_Val_write/1
  ModeAdjust/58(SecRwRtStArmScrnTrgtPos) -> IfVeSMSuSecRwRtStArmScrnTrgtPos_Val_write/1
  modestate32_Val_read/1 -> ModeAdjust/62(modestate32)
  PwrMdChked_Val_read/1 -> ModeAdjust/63(PwrMdChked)
  IfVeSMSbThdRwRtStBkReclnUpwdDnwdMovConfig_Val_read/1 -> ModeAdjust/78(IfVeSMSbThdRwRtStBkReclnUpwdDnwdMovConfig_Val_read)
  IfVeSMSbThdRwRtStCshnFldUpwdDnwdMovConfig_Val_read/1 -> ModeAdjust/79(IfVeSMSbThdRwRtStCshnFldUpwdDnwdMovConfig_Val_read)
  IfVeSMSbThdRwLtStBkReclnUpwdDnwdMovConfig_Val_read/1 -> ModeAdjust/75(IfVeSMSbThdRwLtStBkReclnUpwdDnwdMovConfig_Val_read)
  IfVeSMSbThdRwLtStCshnFldUpwdDnwdMovConfig_Val_read/1 -> ModeAdjust/76(IfVeSMSbThdRwLtStCshnFldUpwdDnwdMovConfig_Val_read)
  IfVeSMSbThdRwLtStFrwdBkwdMovConfig_Val_read/1 -> ModeAdjust/77(IfVeSMSbThdRwLtStFrwdBkwdMovConfig_Val_read)
  IfVeSMSbThdRwRtStFrwdBkwdMovConfig_Val_read/1 -> ModeAdjust/80(IfVeSMSbThdRwRtStFrwdBkwdMovConfig_Val_read)
  IfVeSMSbSecRwRtStLgrstUpwdMovConfig_Val_read/1 -> ModeAdjust/73(IfVeSMSbSecRwRtStLgrstUpwdMovConfig_Val_read)
  IfVeSMSbSecRwRtStLtwdRtwdMovConfig_Val_read/1 -> ModeAdjust/74(IfVeSMSbSecRwRtStLtwdRtwdMovConfig_Val_read)
  IfVeSMSbSecRwRtStBkReclnUpwdDnwdMovConfig_Val_read/1 -> ModeAdjust/70(IfVeSMSbSecRwRtStBkReclnUpwdDnwdMovConfig_Val_read)
  IfVeSMSbSecRwRtStBlstOtwdInwdMovConfig_Val_read/1 -> ModeAdjust/71(IfVeSMSbSecRwRtStBlstOtwdInwdMovConfig_Val_read)
  IfVeSMSbSecRwRtStFrwdBkwdMovConfig_Val_read/1 -> ModeAdjust/72(IfVeSMSbSecRwRtStFrwdBkwdMovConfig_Val_read)
  IfVeSMSbPassStFrwdBkwdMovConfig_Val_read/1 -> ModeAdjust/68(IfVeSMSbPassStFrwdBkwdMovConfig_Val_read)
  IfVeSMSbPassStFtUpwdDnwdMovConfig_Val_read/1 -> ModeAdjust/69(IfVeSMSbPassStFtUpwdDnwdMovConfig_Val_read)
  IfVeSMSbDrvStFrwdBkwdMovConfig_Val_read/1 -> ModeAdjust/65(IfVeSMSbDrvStFrwdBkwdMovConfig_Val_read)
  IfVeSMSbDrvStFtUpwdDnwdMovConfig_Val_read/1 -> ModeAdjust/66(IfVeSMSbDrvStFtUpwdDnwdMovConfig_Val_read)
  IfVeSMSbPassStBkReclnUpwdDnwdMovConfig_Val_read/1 -> ModeAdjust/67(IfVeSMSbPassStBkReclnUpwdDnwdMovConfig_Val_read)
  IfVeSMSbDrvStBkReclnUpwdDnwdMovConfig_Val_read/1 -> ModeAdjust/64(IfVeSMSbDrvStBkReclnUpwdDnwdMovConfig_Val_read)
  IfVeSMSuSecRwLtStLgrstOtwdInwdPos_Val_read/1 -> ModeAdjust/81(IfVeSMSuSecRwLtStLgrstOtwdInwdPos_Val_read)
  IfVeSMSuRrLtStFtUpwdDnwdPos_Val_read/1 -> ModeAdjust/82(IfVeSMSuRrLtStFtUpwdDnwdPos_Val_read)
  IfVeSMSuRrLtStFtUpwdDnwdPosV_Val_read/1 -> ModeAdjust/84(IfVeSMSuRrLtStFtUpwdDnwdPosV_Val_read)
  IfVeSMSuSecRwLtStLgrstOtwdInwdPosV_Val_read/1 -> ModeAdjust/83(IfVeSMSuSecRwLtStLgrstOtwdInwdPosV_Val_read)
  IfVeSMSuSecRwRtStLgrstOtwdInwdPos_Val_read/1 -> ModeAdjust/85(IfVeSMSuSecRwRtStLgrstOtwdInwdPos_Val_read)
  IfVeSMSuRrRtStFtUpwdDnwdPos_Val_read/1 -> ModeAdjust/86(IfVeSMSuRrRtStFtUpwdDnwdPos_Val_read)
  IfVeSMSuRrRtStFtUpwdDnwdPosV_Val_read/1 -> ModeAdjust/88(IfVeSMSuRrRtStFtUpwdDnwdPosV_Val_read)
  IfVeSMSuSecRwRtStLgrstOtwdInwdPosV_Val_read/1 -> ModeAdjust/87(IfVeSMSuSecRwRtStLgrstOtwdInwdPosV_Val_read)
  ModeAdjust/73(isRtLyArrivedAtTargetPos) -> isRtLyArrivedAtTargetPos_Val_write/1
  ModeAdjust/70(isRtFamlyArrivedAtTargetPos) -> isRtFamlyArrivedAtTargetPos_Val_write/1
  ModeAdjust/72(isLfLyArrivedAtTargetPos) -> isLfLyArrivedAtTargetPos_Val_write/1
  ModeAdjust/69(isLfFamlyArrivedAtTargetPos) -> isLfFamlyArrivedAtTargetPos_Val_write/1
  ModeAdjust/71(isINTMArrivedAtTargetPos) -> isINTMArrivedAtTargetPos_Val_write/1
  ModeAdjust/68(isRtLyDoneFailed) -> isRtLyDoneFailed_Val_write/1
  ModeAdjust/67(isRtLyDoneOK) -> isRtLyDoneOK_Val_write/1
  ModeAdjust/66(isLfLyDoneFailed) -> isLfLyDoneFailed_Val_write/1
  ModeAdjust/65(isLfLyDoneOK) -> isLfLyDoneOK_Val_write/1
  ModeAdjust/64(isINTMDoneFailed) -> isINTMDoneFailed_Val_write/1
  ModeAdjust/63(isINTMDoneOK) -> isINTMDoneOK_Val_write/1
  ModeAdjust/62(isRfFamlyDoneFailed) -> isRfFamlyDoneFailed_Val_write/1
  ModeAdjust/61(isRfFamlyDoneOK) -> isRfFamlyDoneOK_Val_write/1
  ModeAdjust/60(isLfFamlyDoneFailed) -> isLfFamlyDoneFailed_Val_write/1
  ModeAdjust/59(isLfFamlyDoneOK) -> isLfFamlyDoneOK_Val_write/1
  ModeAdjust/74(IfVeSMSuRrLtStFtUpwdDnwdTrgtPos_Val_write) -> IfVeSMSuRrLtStFtUpwdDnwdTrgtPos_Val_write/1
  ModeAdjust/75(IfVeSMSuRrRtStFtUpwdDnwdTrgtPos_Val_write) -> IfVeSMSuRrRtStFtUpwdDnwdTrgtPos_Val_write/1
  ModeAdjust/76(IfVeSMSuSecRwLtStLgrstOtwdInwdTrgtPos_Val_write) -> IfVeSMSuSecRwLtStLgrstOtwdInwdTrgtPos_Val_write/1
  ModeAdjust/77(IfVeSMSuSecRwRtStLgrstOtwdInwdTrgtPos_Val_write) -> IfVeSMSuSecRwRtStLgrstOtwdInwdTrgtPos_Val_write/1
  IfVeSMSbSecRwRtSLgrstExpdMovConfig_Val_read/1 -> ModeAdjust/89(IfVeSMSbSecRwRtSLgrstExpdMovConfig_Val_read)
  IfVeSMSbSecRwRtStFtrstMovConfig_Val_read/1 -> ModeAdjust/90(IfVeSMSbSecRwRtStFtrstMovConfig_Val_read)
  IfVeSMSbSecRwRtStHdUpwdDnwdMovConfig_Val_read/1 -> ModeAdjust/91(IfVeSMSbSecRwRtStHdUpwdDnwdMovConfig_Val_read)
  IfVeSMSbThdRwLtStFrwdCmdSrv_Val_read/1 -> ModeAdjust/92(IfVeSMSbThdRwLtStFrwdCmdSrv_Val_read)
  IfVeSMSbThdRwRtStFrwdCmdSrv_Val_read/1 -> ModeAdjust/93(IfVeSMSbThdRwRtStFrwdCmdSrv_Val_read)
  ModeAdjust/79(IfVeSMSuSecRwRtStHdrstFrwdBkwdTrgtPos_Val_write) -> IfVeSMSuSecRwRtStHdrstFrwdBkwdTrgtPos_Val_write/1
  ModeAdjust/78(IfVeSMSuSecRwLtStHdrstFrwdBkwdTrgtPos_Val_write) -> IfVeSMSuSecRwLtStHdrstFrwdBkwdTrgtPos_Val_write/1
  IfVeSMSbSecRwRtStHdrstFrwdBkwdMovConfig_Val_read/1 -> ModeAdjust/94(IfVeSMSbSecRwRtStHdrstFrwdBkwdMovConfig_Val_read)
  IfVeSMSuSecRwLtStHdrstFrwdBkwdPos_Val_read/1 -> ModeAdjust/95(IfVeSMSuSecRwLtStHdrstFrwdBkwdPos_Val_read)
  IfVeSMSuSecRwLtStHdrstFrwdBkwdPosV_Val_read/1 -> ModeAdjust/96(IfVeSMSuSecRwLtStHdrstFrwdBkwdPosV_Val_read)
  IfVeSMSuSecRwRtStHdrstFrwdBkwdPos_Val_read/1 -> ModeAdjust/97(IfVeSMSuSecRwRtStHdrstFrwdBkwdPos_Val_read)
  IfVeSMSuSecRwRtStHdrstFrwdBkwdPosV_Val_read/1 -> ModeAdjust/98(IfVeSMSuSecRwRtStHdrstFrwdBkwdPosV_Val_read)
  IfVeSMSeNotSecRowLeSeaOccStat_Val_read/1 -> ModeAdjust/99(IfVeSMSeNotSecRowLeSeaOccStat_Val_read)
  IfVeSMSeNotSecRowRtSeaOccStat_Val_read/1 -> ModeAdjust/100(IfVeSMSeNotSecRowRtSeaOccStat_Val_read)
  ModeAdjust/95(IfVeSMSeSecRwLtStMdRclLgSldSpdCrl_Val_write) -> IfVeSMSeSecRwLtStMdRclLgSldSpdCrl_Val_write/1
  ModeAdjust/96(IfVeSMSeSecRwRtStMdRclLgSldSpdCrl_Val_write) -> IfVeSMSeSecRwRtStMdRclLgSldSpdCrl_Val_write/1
  ModeAdjust/97(IfVeSMSeThdRwLtStMdRclLgSldSpdCrl_Val_write) -> IfVeSMSeThdRwLtStMdRclLgSldSpdCrl_Val_write/1
  ModeAdjust/98(IfVeSMSeThdRwRtStMdRclLgSldSpdCrl_Val_write) -> IfVeSMSeThdRwRtStMdRclLgSldSpdCrl_Val_write/1
  ModeAdjust/80(isINTMRArrivedAtTargetPos) -> isINTMRArrivedAtTargetPos_Val_write/1
  ModeAdjust/86(isINTMRDoneFailed) -> isINTMRDoneFailed_Val_write/1
  ModeAdjust/85(isINTMRDoneOK) -> isINTMRDoneOK_Val_write/1
  ModeAdjust/83(isLgrstCloseLArrivedAtTargetPos) -> isLgrstCloseLArrivedAtTargetPos_Val_write/1
  ModeAdjust/92(isLgrstCloseLDoneFailed) -> isLgrstCloseLDoneFailed_Val_write/1
  ModeAdjust/91(isLgrstCloseLDoneOK) -> isLgrstCloseLDoneOK_Val_write/1
  ModeAdjust/84(isLgrstCloseRArrivedAtTargetPos) -> isLgrstCloseRArrivedAtTargetPos_Val_write/1
  ModeAdjust/94(isLgrstCloseRDoneFailed) -> isLgrstCloseRDoneFailed_Val_write/1
  ModeAdjust/93(isLgrstCloseRDoneOK) -> isLgrstCloseRDoneOK_Val_write/1
  ModeAdjust/81(isLgrstOpenLArrivedAtTargetPos) -> isLgrstOpenLArrivedAtTargetPos_Val_write/1
  ModeAdjust/88(isLgrstOpenLDoneFailed) -> isLgrstOpenLDoneFailed_Val_write/1
  ModeAdjust/87(isLgrstOpenLDoneOK) -> isLgrstOpenLDoneOK_Val_write/1
  ModeAdjust/82(isLgrstOpenRArrivedAtTargetPos) -> isLgrstOpenRArrivedAtTargetPos_Val_write/1
  ModeAdjust/90(isLgrstOpenRDoneFailed) -> isLgrstOpenRDoneFailed_Val_write/1
  ModeAdjust/89(isLgrstOpenRDoneOK) -> isLgrstOpenRDoneOK_Val_write/1
  IfVeSMSeStNumConfig_Val_read/1 -> ModeAdjust/101(IfVeSMSeStNumConfig_Val_read)

== system ModeAdjust/ModeAdjust_Init ==
  Event Listener : EventListener  EventName=reset
